simulink model "EKF"  (R2019a)
settings: Solver=VariableStepAuto  StartTime=0.0  StopTime=10.0  RelTol=1e-3
values from neighbouring files (symbols this model uses):
  Ts = 4e-3    (= 0.004)    [IMU_init.m]
undefined symbols (not defined in the file or in its folder): Jx, Jy, Jz, m
settings Model: Creator=matte  LastModifiedBy=david
settings DataIOCC: ReturnWorkspaceOutputs=off
settings DebuggingCC: UnderSpecifiedDimensionMsg=error  ArithmeticOperatorsInVariantConditions=warning
settings SFSimCC: SimUseLocalCustomCode=off
settings RTWCC: RTWUseLocalCustomCode=off
settings CodeAppCC: StateflowObjectComments=on

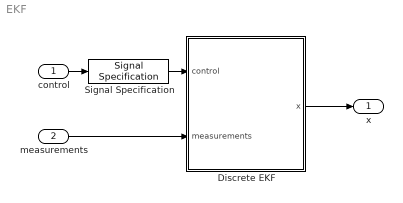
== system EKF ==
  control : Inport
  measurements : Inport  Port=2
  Discrete EKF : Subsystem
  Signal Specification : SignalSpecification  Dimensions=4
  x : Outport
  wires:
  control/1 -> Signal Specification/1
  measurements/1 -> Discrete EKF/2(measurements)
  Discrete EKF/1(x) -> x/1
  Signal Specification/1 -> Discrete EKF/1(control)

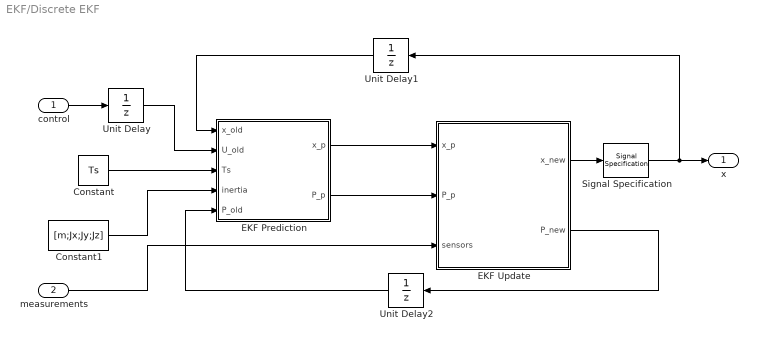
== system EKF/Discrete EKF ==
  control : Inport
  measurements : Inport  Port=2
  Constant : Constant  Value=Ts
  Constant1 : Constant  Value=[m;Jx;Jy;Jz]
  EKF Prediction : MATLAB Function  TreatAsAtomicUnit=on
  EKF Update : MATLAB Function  TreatAsAtomicUnit=on
  Signal Specification : SignalSpecification  Dimensions=10
  Unit Delay : UnitDelay  SampleTime=-1  HasFrameUpgradeWarning=on
  Unit Delay1 : UnitDelay  SampleTime=-1  HasFrameUpgradeWarning=on
  Unit Delay2 : UnitDelay  SampleTime=-1  HasFrameUpgradeWarning=on
  x : Outport
  wires:
  control/1 -> Unit Delay/1
  Unit Delay1/1 -> EKF Prediction/1(x_old)
  Unit Delay2/1 -> EKF Prediction/5(P_old)
  measurements/1 -> EKF Update/3(sensors)
  EKF Update/1(x_new) -> Signal Specification/1
  Unit Delay/1 -> EKF Prediction/2(U_old)
  EKF Prediction/2(P_p) -> EKF Update/2(P_p)
  EKF Update/2(P_new) -> Unit Delay2/1
  Constant/1 -> EKF Prediction/3(Ts)
  Constant1/1 -> EKF Prediction/4(inertia)
  EKF Prediction/1(x_p) -> EKF Update/1(x_p)
  Signal Specification/1 -> Unit Delay1/1, x/1

== matlab function EKF/Discrete EKF/EKF Update ==
  data: x_p input; P_p input; x_new output; sensors input; P_new output
function [x_new,P_new] = update(x_p,P_p,sensors)
%--------------------------------------------------------------------------
% Author: Matteo Scanavino (matteo.scanavino@polito.it)
% Affiliation: Politecnico di Torino - Department of Mechanical and
% Aerospace Engineering (DIMEAS)
% Year: 2019
% -------------------------------------------------------------------------
% 
% This script performs the prediction step of the extended kalman filter
% 
% Input:    x_p       ->  state vector prediction              
%           P_p       ->  covariance matrix prediction
%           sensors   ->  sensor data    
% Output:   x_new     ->  state vector update 
%           P_new     ->  covariance matrix update
%           K         ->  kalman gain
%--------------------------------------------------------------------------
%
IMU_init; 
%--------------------------------------------------------------------------
% State variable
%--------------------------------------------------------------------------
% Linear velocity
u       = x_p(1);
v       = x_p(2); 
w       = x_p(3); 
%
% Angular velocity
p       = x_p(4); 
q       = x_p(5) ;
r       = x_p(6); 
%
% Euler angles
phi     = x_p(7); 
theta   = x_p(8); 
psi     = x_p(9); 
%
% Altitude 
z       = x_p(10); 
%
% Rotation matrix (form ned to body)
R       =   [cos(theta)*cos(psi)                               ...
             cos(theta)*sin(psi)                               ...       
             -sin(theta);                                      ...
             -cos(phi)*sin(psi)+sin(phi)*sin(theta)*cos(psi)   ...
             cos(phi)*cos(psi)+sin(phi)*sin(theta)*sin(psi)    ...
             sin(phi)*cos(theta);                              ...
             sin(phi)*sin(psi)+cos(phi)*sin(theta)*cos(psi)    ...
             -sin(phi)*cos(psi)+cos(phi)*sin(theta)*sin(psi)   ...
             cos(phi)*cos(theta)];
%
%--------------------------------------------------------------------------
% Sensor equations
%--------------------------------------------------------------------------
% Accelerometer
ya      = Ma*[r*v - q*w; p*w - r*u; q*u - p*v+U(1)/m] + ba; 
%
% Gyroscope
yg      = Mg*[p;q;r] + bg;
%
% Magnetometer
ym      = Mm*R*mag + bm; 
%
% Barometer
yb      = kb*P0*exp(-(g*z)/(Ra*T0)) + bb; 
%
% −−−−−−−−−−−−−−−−−−−−−−−−−−−−−−−−−−−−−−−−−−−−−−−−−−−−--------
% Partial derivatives of the rotation matrix
% with respect to phi, theta and psi
% −−−−−−−−−−−−−−−−−−−−−−−−−−−−−−−−−−−−−−−−−−−−−−−−−−−−--------
Rdphi = [ 0 , 0 , 0 ;
         cos(psi)*sin(theta)*cos(phi) + sin(psi)*sin(phi), ...
         sin(psi)*sin(theta)*cos(phi) - cos(psi)*sin(phi), ...
         cos(theta)*cos(psi);
         -cos(psi)*sin(theta)*sin(phi) + sin(psi)*cos(phi), ...
         -sin(psi)*sin(theta)*sin(phi) - cos(psi)*cos(phi), ...
         -cos(theta)*sin(phi)];
%
Rdtheta = [-cos(psi)*sin(theta), ...
           -sin(psi)*sin(theta), ...
           -cos(theta);
           cos(psi)*cos(theta)*sin(phi), ...
           sin(psi)*cos(theta)*sin(phi), ...
           -sin(theta)*sin(phi);
           cos(psi)*cos(theta)*cos(phi), ...
           sin(psi)*cos(theta)*cos(phi), ...
           -sin(theta)*cos(phi)] ;
%
Rdpsi = [ -sin(psi)*cos(theta),cos(psi)*cos(theta),0;
          -sin(psi)*sin(theta)*sin(phi) - cos(psi)*cos(phi), ...
          cos(psi)*sin(theta)*sin(phi)- sin(psi)*cos(phi), 0;
          -sin(psi)*sin(theta)*cos(phi) + cos(psi)*sin(phi), ...
          cos(psi)*sin(theta)*cos(phi) + sin(psi)*sin(phi), 0] ;
%
% −−−−−−−−−−−−−−−−−−−−−−−−−−−−−−−−−−−−−−−−−−−−−−−−−−−−--------
% Jacobian of the sensor equations 
% −−−−−−−−−−−−−−−−−−−−−−−−−−−−−−−−−−−−−−−−−−−−−−−−−−−−--------
% Accelerometer
J1 = Ma*[0 r -q ; -r 0 p ; q -p 0 ] ;
J2 = Ma*[0 -w v ; w 0 -u ; -v u 0 ] ;
% Magnetometer
J3 = [Mm*Rdphi*mf_e Mm*Rdtheta*mf_e Mm*Rdpsi*mf_e ] ;
%
% Altimete r
Ja = -(kb*P0*g)/(Ra*T0)*exp(-(g*z)/(Ra*T0));
%
% Final matrix
H = zeros(10) ;
H(1:3,1:3) = J1 ;
H(1:3,4:6) = J2 ;
H(4:6,4:6) = Mg;
H(7:9,7:9) = J3 ;
H(10,10) = Ja ;
%
%---------−−−−−−−−−−−−−−−−−−−−−−−−−−−−−−−−−−−−−−−−−−−−−−−−−−−−
% State update
%---------−−−−−−−−−−−−−−−−−−−−−−−−−−−−−−−−−−−−−−−−−−−−−−−−−−−−
% Measurement residual
y_res = sensors - [ ya ; yg ; ym; yb ];
% Innovation cova rian c e
S = H*P_p*H' + R_e;
%
% Kalman gain
K = P_p*H' / S ;
%
% Updated state estimate
x_new = x_p + K*y_res ;
% Updated e stimated covariance
P_new = ( eye (10) - H*K) *P_p;
%
end

== matlab function EKF/Discrete EKF/EKF Prediction ==
  data: x_old input; U_old input; Ts input; inertia input; x_p output; P_old input; P_p output
function [x_p,P_p] = prediction(x_old,U_old,Ts,inertia,P_old)
%--------------------------------------------------------------------------
% Author: Matteo Scanavino (matteo.scanavino@polito.it)
% Affiliation: Politecnico di Torino - Department of Mechanical and
% Aerospace Engineering (DIMEAS)
% Year: 2019
% -------------------------------------------------------------------------
% 
% This script performs the prediction step of the extended kalman filter
% 
% Input:    x_old   ->  state vector at previous time step              
%           P_old   ->  covariance matrix at previous time step
%           u_old   ->  control vector at previous time step    
% Output:   x_p     ->  state vector prediction 
%           P_p     -> covariance matrix prediction
%
%--------------------------------------------------------------------------
g           = 9.81;                 % Gravity   [m/s^2]
m           = inertia(1);           % Mass      [kg]
Ix          = inertia(2);           % Ix
Iy          = inertia(3);           % Iy
Iz          = inertia(4);           % Iz
Q_e = 0.01*eye(10);
%--------------------------------------------------------------------------
% State variables
%--------------------------------------------------------------------------
% Linear velocity 
u_old       = x_old(1); 
v_old       = x_old(2); 
w_old       = x_old(3); 
%
% Angular velocity
p_old       = x_old(4); 
q_old       = x_old(5); 
r_old       = x_old(6); 
%    
% Euler angle
phi_old     = x_old(7); 
theta_old   = x_old(8); 
psi_old     = x_old(9); 
%
%--------------------------------------------------------------------------
% State prediction 
%--------------------------------------------------------------------------
d_x    =  zeros(10,1); 
d_x(1) =  r_old*v_old - q_old*w_old + g*sin(theta_old); %u
d_x(2) = -r_old*u_old + p_old*w_old - g*cos(theta_old)*sin(phi_old); %v  
d_x(3) =  q_old*u_old - p_old*v_old - g*cos(theta_old)*cos(phi_old) + ...
          U_old(1) / m; %w
d_x(4) = (Iy - Iz)*q_old*r_old/(Ix) + U_old(2)/Ix; %p
d_x(5) = (Iz - Ix)*p_old*r_old/(Iy) + U_old(3)/Iy; %q
d_x(6) = (Ix - Iy)*p_old*q_old/(Iz) + U_old(4)/Iz; %r
d_x(7) = p_old + sin(phi_old)*tan(theta_old)*q_old + ...
         cos(phi_old)*tan(theta_old)*r_old; %phi
d_x(8) = cos(phi_old)*q_old - sin(phi_old)*r_old; %theta
d_x(9) = (sin(phi_old)*q_old)/cos(theta_old) + ...
         (cos(phi_old)*r_old)/cos(theta_old); %psi
d_x(10)= -sin(theta_old)*u_old - cos(theta_old)*sin(phi_old)*v_old + ...
        cos(theta_old)*cos(phi_old)*w_old; %z
%    
x_p    = x_old + Ts*d_x; 
%   
%--------------------------------------------------------------------------
% Covariance prediction 
%--------------------------------------------------------------------------
% Partial derivatives of the state equations
F_old       = eye(10); 
F_old(1,2)  = r_old; 
F_old(1,3)  = -q_old; 
F_old(1,5)  = -w_old; 
F_old(1,6)  = v_old; 
F_old(1,8)  = g*cos(theta_old); 
F_old(2,1)  = -r_old; 
F_old(2,3)  = p_old; 
F_old(2,4)  = w_old; 
F_old(2,6)  = -u_old; 
F_old(2,7)  = -g*cos(theta_old)*cos(phi_old); 
F_old(2,8)  = g*sin(theta_old)*sin(phi_old); 
F_old(3,1)  = q_old;
F_old(3,2)  = -p_old; 
F_old(3,4)  = -v_old; 
F_old(3,5)  = u_old; 
F_old(3,7)  = g*cos(theta_old)*sin(phi_old); 
F_old(3,8)  = g*sin(theta_old)*cos(phi_old); 
F_old(4,5)  = (Iy - Iz)*r_old/Ix; 
F_old(4,6)  = (Iy - Iz)*q_old/Ix; 
F_old(5,4)  = (Iz - Ix)*r_old/Iy; 
F_old(5,6)  = (Iz - Ix)*p_old/Iy; 
F_old(6,4)  = (Ix - Iy)*q_old/Iz; 
F_old(6,5)  = (Ix - Iy)*p_old/Iz; 
F_old(7,4)  = 1; 
F_old(7,5)  = sin(phi_old)*tan(theta_old); 
F_old(7,6)  = cos(phi_old)*tan(theta_old); 
F_old(7,7)  = 1 + cos(phi_old)*tan(theta_old)*q_old - ...
              sin(phi_old)*cos(theta_old)*q_old; 
F_old(7,8)  = (sin(phi_old)*q_old + cos(phi_old)*r_old) / cos(theta_old)^2;
F_old(8,5) = cos(phi_old);
F_old(8,6) = -sin(phi_old);
F_old(8,7) = -cos(phi_old)*r_old - sin(phi_old)*q_old;
F_old(9,5) = sin(phi_old)/cos(theta_old);
F_old(9,6) = cos(phi_old)/cos(theta_old) ;
F_old(9,7) = (cos(phi_old)*q_old - sin(phi_old)*r_old)/cos(theta_old);
F_old(9,8) = sin(theta_old)*(sin(phi_old)*r_old + ...
             cos(phi_old)*q_old)/cos(theta_old)^2;
F_old(10,1)= -sin(theta_old);
F_old(10,2)= cos(theta_old)*sin(phi_old);
F_old(10,3)= cos(theta_old)*cos(phi_old);
F_old(10,7)= cos(theta_old)*cos(phi_old)*v_old - ...
             cos(theta_old)*sin(phi_old)*w_old;
F_old(10,8)= -cos(theta_old)*u_old - sin(theta_old)*sin(phi_old)*v_old ...
             -cos(theta_old)*sin(theta_old)*w_old;
% 
F_old = Ts*F_old; 
%
% Covariance matrix update
P_p = F_old*P_old*F_old' + Q_e;
%
end
